simulink model "sml_unicycle"  (R2016a)
settings: Solver=VariableStepAuto  StartTime=0.0  StopTime=10.0  RelTol=1e-3
libraries: simulink x1
settings Model: Creator=Duy Nam  LastModifiedBy=Duy Nam

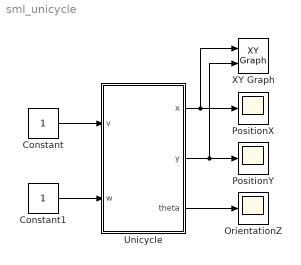
== system sml_unicycle ==
  Constant : Constant
  Constant1 : Constant
  OrientationZ : Scope
  PositionX : Scope
  PositionY : Scope
  Unicycle : Subsystem
  XY Graph : simulink/Sinks/XY Graph  xmin=0  xmax=10  ymin=0  ymax=10  st=-1
  wires:
  Unicycle/1(x) -> XY Graph/1, PositionX/1
  Unicycle/2(y) -> XY Graph/2, PositionY/1
  Unicycle/3(theta) -> OrientationZ/1
  Constant/1 -> Unicycle/1(v)
  Constant1/1 -> Unicycle/2(w)

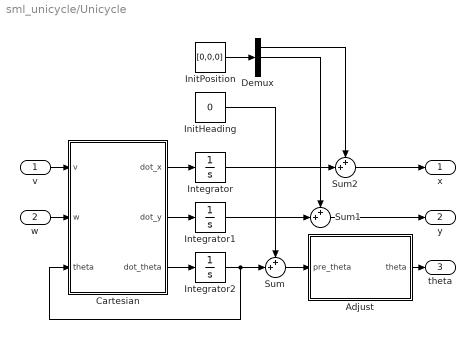
== system sml_unicycle/Unicycle ==
  v : Inport
  w : Inport  Port=2
  Adjust : MATLAB Function  TreatAsAtomicUnit=on
  Cartesian : MATLAB Function  TreatAsAtomicUnit=on
  Demux : Demux  Outputs=3
  InitHeading : Constant  Value=0
  InitPosition : Constant  Value=[0,0,0]
  Integrator : Integrator
  Integrator1 : Integrator
  Integrator2 : Integrator
  Sum : Sum  Inputs=++|
  Sum1 : Sum  Inputs=++|
  Sum2 : Sum  Inputs=++|
  x : Outport
  y : Outport  Port=2
  theta : Outport  Port=3
  wires:
  Cartesian/2(dot_y) -> Integrator1/1
  Cartesian/1(dot_x) -> Integrator/1
  Cartesian/3(dot_theta) -> Integrator2/1
  Integrator2/1 -> Sum/2, Cartesian/3(theta)
  Adjust/1(theta) -> theta/1
  Integrator1/1 -> Sum1/2
  Integrator/1 -> Sum2/2
  v/1 -> Cartesian/1(v)
  w/1 -> Cartesian/2(w)
  Sum/1 -> Adjust/1(pre_theta)
  Sum1/1 -> y/1
  Sum2/1 -> x/1
  InitHeading/1 -> Sum/1
  InitPosition/1 -> Demux/1
  Demux/1 -> Sum2/1
  Demux/2 -> Sum1/1

== matlab function sml_unicycle/Unicycle/Adjust ==
  data: pre_theta input; theta output
function theta = Adjust(pre_theta)
% ADJUST adjust the orientation z of robot is always between (-pi/2;pi/2)
%% INPUTS
% pre_theta = The orientation Z before adjust
%% OUTPUTS
% theta = The orientation Z after adjust
%% Adjust
theta = pre_theta - 2*pi*floor((pre_theta + pi)/(2*pi));
end

== matlab function sml_unicycle/Unicycle/Cartesian ==
  data: v input; dot_x output; w input; theta input; dot_y output; dot_theta output
function [dot_x, dot_y, dot_theta] = Cartesian(v, w, theta)
% CARTESIAN Convert robot frame to the world frame
%% INPUTS
% v     = The linear velocity of Robot
% w     = The angular velocity of Robot
% theta = The heading angular of robot in world frame
%% OUTPUTS
% dot_x = The linear x velocity in world frame
% dot_y = The linear y velocity in world frame
% dot_theta = The angular z velocity in world frame
%% Castesian
dot_x = v*cos(theta);
dot_y = v*sin(theta);
dot_theta = w;
end
